simulink subsystem "Controller_HVAC"  (R2024b)
settings: Solver=VariableStepAuto  StartTime=0.0  StopTime=10.0  RelTol=1e-3
undefined symbols (not defined in the file or in its folder): battery, vehicle
libraries: slpidlib x3, BatteryCurrentManagement x2
(part 2 of 2)

== system Controller_HVAC/Vehicle Control/Torque Control/Brake//Motor Trq Split/Braking Torque ==
  BrkFac : Inport
  MaxChgTq : Inport  Port=2
  BrkTq : Inport  Port=3
  Add1 : Sum  Inputs=-+
  Max : MinMax  Function=max  Inputs=2
  Product : Product
  MechBrkTq : Outport
  RegenBrkTq : Outport  Port=2
  wires:
  BrkFac/1 -> Product/1
  Product/1 -> Max/2
  BrkTq/1 -> Product/2, Add1/2
  Max/1 -> Add1/1, RegenBrkTq/1
  MaxChgTq/1 -> Max/1
  Add1/1 -> MechBrkTq/1

== system Controller_HVAC/Vehicle Control/Torque Control/Charge//Discharge Limit/Unit Conversion ==
  rpm : Inport
  Add : Sum
  Constant : Constant
  Constant6 : Constant
  Product1 : Product
  Signal Specification : SignalSpecification  OutMin=[0]  Unit=rad/sec
  Unit Conversion : UnitConversion
  rad/s : Outport
  wires:
  Constant/1 -> Product1/1
  rpm/1 -> Unit Conversion/1
  Unit Conversion/1 -> Signal Specification/1
  Add/1 -> Product1/2
  Product1/1 -> rad/s/1
  Constant6/1 -> Add/2
  Signal Specification/1 -> Add/1

== stateflow chart Controller_HVAC/Vehicle Control/Torque Control/Trq Split Fac/Stateflow ==
  state FrontWheel
    Mode=0;
    TrqEm1Fac=1;
    TrqEm2Fac=0;
  state BrakeDistr
    Mode=2;
    TrqEm1Fac=1;
  state AWD
    Mode=1;
    TrqEm1Fac=0.6;
    TrqEm2Fac=0.4;
  (default) -> FrontWheel
  FrontWheel -> BrakeDistr [order 2] : [Tq<=0]
  BrakeDistr -> FrontWheel : [Tq>0]
  AWD -> FrontWheel : [Tq<10 | AWDstate ==0]
  FrontWheel -> AWD [order 1] : [Tq>100 & AWDstate==1]
  data: Tq input; Mode output; TrqEm2Fac output; TrqEm1Fac output; AWDstate input
